simulink model "off_grid_NPC"  (R2015b)
settings: Solver=ode23tb  StartTime=0.0  StopTime=4  RelTol=1e-3
PreLoadFcn:
  | load  power_3levelVSC.mat
  | Ts_Power=5e-6;
  | Ts_Control=100e-6;
undefined symbols (not defined in the file): DiscIntNeverNeededParam
libraries: powerlib x25, powerlib_meascontrol x18, powerlib_extras x6, simulink x6, simulink_extras x1
settings Model: Creator=Pouyan  LastModifiedBy=fujitsu
settings DataIOCC: SaveFormat=Array  SignalLoggingSaveFormat=ModelDataLogs
settings OptimizationCC: ExpressionDepthLimit=2147483647
settings DebuggingCC: UnderspecifiedInitializationDetection=Classic  MergeDetectMultiDrivingBlocksExec=none  SolverPrmCheckMsg=warning  FcnCallInpInsideContextMsg=UseLocalSettings  StateNameClashWarn=warning
settings HardwareCC: ProdBitPerPointer=32  ProdLargestAtomicFloat=None  ProdIntDivRoundTo=Undefined  ProdEndianess=Unspecified  ProdWordSize=32  ProdHWDeviceType=32-bit Generic
settings GRTTargetCC: GeneratePreprocessorConditionals=Disable all  CombineOutputUpdateFcns=off  GRTInterface=on
settings ConfigComp: CovModelRefEnable=Off

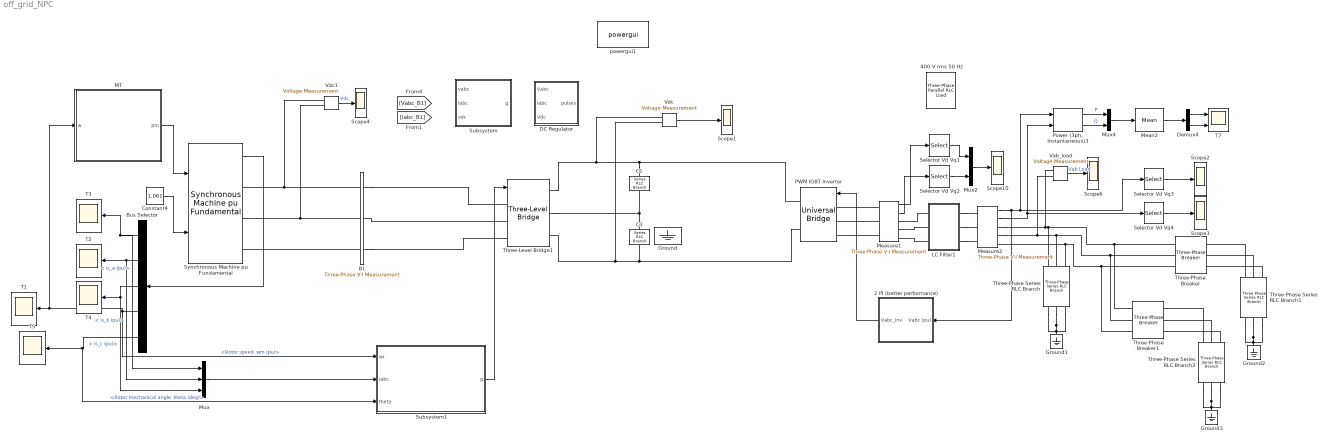
== system off_grid_NPC ==
  " 400 V rms 50 Hz" : powerlib/Elements/Three-Phase Parallel RLC Load  LConnTagsString=A|B|C  Configuration=Y (grounded)  NominalVoltage=400  Vabc=[1e3 1e3 1e3]  Vabcp=[1e3 1e3 1e3]  NominalFrequency=50  UnbalancedPower=off  ActivePower=50e3  InductivePower=0  CapacitivePower=0  Pabc=[10e3 9e3 11e3]  QLabc=[100 90 110]  QCabc=[100 90 110]  Pabcp=[10e3 9e3 11e3]  QLabcp=[100 90 110]  QCabcp=[100 90 110]  Measurements=None  LoadType=constant Z
  2 PI (better performance) : Subsystem  mask{kp=0.01, ki=5}
  B1 : powerlib/Measurements/Three-Phase V-I Measurement  VoltageMeasurement=phase-to-ground  SetLabelV=on  LabelV=Vabc_B1  Vpu=off  VpuLL=off  CurrentMeasurement=yes  SetLabelI=on  LabelI=Iabc_B1  Ipu=off  Pbase=100e6  Vbase=500e3  OutputType=Magnitude  PhasorSimulation=off  PSBequivalent=0
  Bus Selector : BusSelector  OutputSignals="Stator current. is_a (pu),Stator current. is_b (pu),Stator current. is_c (pu),Mechanical.Rotor speed  wm (pu),Mechanical.Rotor mechanical angle  theta (deg)"
  C1 : powerlib/Elements/Series RLC Branch  LConnTagsString=__new0  RConnTagsString=__new0  BranchType=C  Resistance=1.0  Inductance=1.0  SetiL0=off  InitialCurrent=0  Capacitance=75000e-06  Setx0=off  InitialVoltage=0  Measurements=None
  C3 : powerlib/Elements/Series RLC Branch  LConnTagsString=__new0  RConnTagsString=__new0  BranchType=C  Resistance=1.0  Inductance=1.0  SetiL0=off  InitialCurrent=0  Capacitance=75000e-06  Setx0=off  InitialVoltage=0  Measurements=None
  Constant4 : Constant  Value=1.061
  DC Regulator : Subsystem  mask(DC Voltage Regulator){Vdc_Ref=750}
      mask prompts: Vdc_Ref "DC voltage setpoint (V):"
  Demux4 : Demux  Outputs=2
  Ground{,1..3} (4 alike) : powerlib/Elements/Ground  LConnTagsString=a
  LC Filter1 : Subsystem
  MT : Subsystem
  Mean2 : powerlib_meascontrol/Measurements/Mean  Freq=50  Vinit=0  Ts=50e-6
  Measure1 : powerlib/Measurements/Three-Phase V-I Measurement  VoltageMeasurement=phase-to-phase  SetLabelV=off  LabelV=V1  Vpu=off  VpuLL=off  CurrentMeasurement=yes  SetLabelI=off  LabelI=I1  Ipu=off  Pbase=10e3  Vbase=400  OutputType=Magnitude  PhasorSimulation=off  PSBequivalent=0
  Measure2 : powerlib/Measurements/Three-Phase V-I Measurement  VoltageMeasurement=phase-to-phase  SetLabelV=off  LabelV=V1  Vpu=off  VpuLL=on  CurrentMeasurement=yes  SetLabelI=off  LabelI=I1  Ipu=on  Pbase=20e3  Vbase=400  OutputType=Magnitude  PhasorSimulation=off  PSBequivalent=0
  Mux : Mux  Inputs=3
  Mux2 : Mux  Inputs=2
  Mux4 : Mux  Inputs=2
  PWM IGBT Inverter : powerlib/Power Electronics/Universal Bridge  Arms=3  SnubberResistance=5000  SnubberCapacitance=inf  Device=IGBT / Diodes  Ron=1e-3  Lon=0  ForwardVoltages="[  0.0  0.0  ]"  ForwardVoltage=.8  GTOparameters=[ 1e-6 ,1e-6 ]  IGBTparameters=[ 1e-6 , 2e-6 ]  Measurements=Device currents  Measurements_2=None  converterType=Rectifier
  "Power (3ph, Instantaneous)3" : powerlib_meascontrol/Measurements/Power (3ph, Instantaneous)
  Scope{1..4,6,10} (6 alike) : Scope
  Selector Vd Vq{1..4} (4 alike) : Selector  InputPortWidth=3  IndexOptions=Index vector (dialog)  Indices=[1]  OutputSizes=1
  Subsystem : Subsystem  mask{kp=1, ki=5, dcref=750}
      mask prompts: dcref "Vdc_ref"
  Subsystem1 : Subsystem  mask{kp=1, ki=5}
  Synchronous Machine pu Fundamental : powerlib/Machines/Synchronous Machine pu Fundamental  PresetModel=No  MechanicalLoad=Mechanical power Pm  ShowDetailedParameters=on  RotorType=Salient-pole  Units=per unit fundamental parameters  MeasurementBus=off  NominalParameters="[ 60e3  500 1600]"  Stator="[ 0.2503  0.114  0.6875  0.6875 ]"  Field="[ 1  10e15/(100*pi)]"  Dampers2=[0.0652, 0.5134, 0.0287, 0.2553, 7.765e-3, 0.9167 ]  Dampers1="[ 1.17E-02  0.182  1.97E-02  0.384 ]"  Mechanical=[ 6 0 2]  PolePairs=20  InitialConditions="[ 0  0  0  0  0  0  0  0  1 ]"  SetSaturation=off  Saturation=[0.6404,0.7127,0.8441,0.9214,0.9956,1.082,1.19,1.316,1.457;0.7,0.7698,0.8872,0.9466,0.9969,1.046,1.1,1.151,1.201]  LoadFlowParameters=[1,0,0,0,0]  TsPowergui=0  TsBlock=-1  IterativeModel=Trapezoidal non iterative  BusType=swing  Pref=0  Qref=0  Qmin=-inf  Qmax=inf  PLF=0  QLF=0
  T{1..5} (5 alike) : Scope
  T7 : Scope  NumInputPorts=2
  Three-Level Bridge1 : powerlib/Power Electronics/Three-Level Bridge  Arms=3  SnubberResistance=100  SbubberCapacitance=1e-6  Device=IGBT / Diodes  Ron=1e-3  ForwardVoltages=[370 1]  Measurements=All voltages and currents
  Three-Phase Series RLC Branch : powerlib/Elements/Three-Phase Series RLC Branch  LConnTagsString=A|B|C  RConnTagsString=A|B|C  BranchType=R  Resistance=400^2/20000  Inductance=1e-3  Capacitance=1e-6  Measurements=None
  Three-Phase Series RLC Branch1 : powerlib/Elements/Three-Phase Series RLC Branch  LConnTagsString=A|B|C  RConnTagsString=A|B|C  BranchType=R  Resistance=400^2/10000  Inductance=1e-3  Capacitance=1e-6  Measurements=None
  Three-Phase Series RLC Branch2 : powerlib/Elements/Three-Phase Series RLC Branch  LConnTagsString=A|B|C  RConnTagsString=A|B|C  BranchType=R  Resistance=400^2/20000  Inductance=1e-3  Capacitance=1e-6  Measurements=None
  Three-Phase Breaker : powerlib/Elements/Three-Phase Breaker  InitialState=open  SwitchA=on  SwitchB=on  SwitchC=on  SwitchTimes=[1 3]  External=off  BreakerResistance=0.01  SnubberResistance=1e6  SnubberCapacitance=inf  Measurements=None
  Three-Phase Breaker1 : powerlib/Elements/Three-Phase Breaker  InitialState=open  SwitchA=on  SwitchB=on  SwitchC=on  SwitchTimes=[2]  External=off  BreakerResistance=0.01  SnubberResistance=1e6  SnubberCapacitance=inf  Measurements=None
  Vab_load : powerlib/Measurements/Voltage Measurement  Tag=PoWeRsYsTeMmEaSuReMeNt  PhasorSimulation=off  OutputType=Magnitude  PSBequivalent=0
  "Vdc " : powerlib/Measurements/Voltage Measurement  Tag=PoWeRsYsTeMmEaSuReMeNt  PhasorSimulation=off  OutputType=Magnitude  PSBequivalent=0
  Vdc1 : powerlib/Measurements/Voltage Measurement  Tag=PoWeRsYsTeMmEaSuReMeNt  PhasorSimulation=off  OutputType=Magnitude  PSBequivalent=0
  powergui1 : powerlib/powergui  Priority=2  SimulationMode=Discrete  SolverType=Tustin/Backward Euler (TBE)  SampleTime=Ts_Power  frequency=60  SPID=off  DisableSnubberDevices=off  DisableRonSwitches=off  DisableVfSwitches=off  SwTol=0  DisplayEquations=off  Interpol=off  ExternalGateDelay=off  methode=off  Ts=0  FunctionMessages=off  echomessages=off  HookPort=off  EnableUseOfTLC=off  x0status=blocks  frequencyindice=0  Pbase=100e6  ErrMax=1e-4  Iterations=50  UnitsV=kV  UnitsW=MW  buscounter=0  RestoreLinks=warning  ResistiveCurrentMeasurement=off  Frange=logspace(0,3,50)  Ylog=off  Xlog=off  ShowGrid=off  save=off  variable=ZData  structure=VaIa  ZoomFFT=on  StartTime=0.2  cycles=2  DisplayStyle=1  fundamental=60  FreqAxis=off  MaxFrequency=1000  frequencyindicesteady=1  RmsSteady=2  display=off
  wires:
  Vab_load/1 -> Scope6/1  "Vab Load"
  Mux4/1 -> Mean2/1
  Mean2/1 -> Demux4/1
  "Power (3ph, Instantaneous)3"/1 -> Mux4/1  "P"
  "Power (3ph, Instantaneous)3"/2 -> Mux4/2  "Q"
  Demux4/1 -> T7/1
  Demux4/2 -> T7/2
  "Vdc "/1 -> Scope1/1
  MT/1(pm) -> Synchronous Machine pu Fundamental/1
  Synchronous Machine pu Fundamental/1 -> Bus Selector/1
  Bus Selector/4 -> Subsystem1/1(wr), MT/1(w), T1/1  "<Rotor speed  wm (pu)>"
  Constant4/1 -> Synchronous Machine pu Fundamental/2
  Vdc1/1 -> Scope4/1  "Vdc"
  Mux2/1 -> Scope10/1
  Measure1/1 -> Selector Vd Vq1/1
  Selector Vd Vq1/1 -> Mux2/1
  Measure1/2 -> Selector Vd Vq2/1
  Selector Vd Vq2/1 -> Mux2/2
  Measure2/1 -> 2 PI (better performance)/1(Vabc (pu)), "Power (3ph, Instantaneous)3"/1, Selector Vd Vq3/1
  Measure2/2 -> "Power (3ph, Instantaneous)3"/2, Selector Vd Vq4/1
  Selector Vd Vq3/1 -> Scope2/1
  Selector Vd Vq4/1 -> Scope3/1
  2 PI (better performance)/1(Vabc_inv) -> PWM IGBT Inverter/1
  Bus Selector/1 -> Mux/1, T3/1  "< is_a (pu)>"
  Bus Selector/2 -> T2/1, Mux/2  "< is_b (pu)>"
  Bus Selector/3 -> Mux/3, T4/1  "< is_c (pu)>"
  Bus Selector/5 -> Subsystem1/3(theta), T5/1  "<Rotor mechanical angle  theta (deg)>"
  Mux/1 -> Subsystem1/2(iabc)
  Subsystem1/1(g) -> Three-Level Bridge1/1
  connections:
  Measure2/RConn2 -- Three-Phase Breaker1/LConn2 -- Three-Phase Breaker/LConn2 -- Three-Phase Series RLC Branch/LConn2 -- Vab_load/LConn2
  Measure2/RConn1 -- Three-Phase Breaker1/LConn1 -- Three-Phase Breaker/LConn1 -- Three-Phase Series RLC Branch/LConn1 -- Vab_load/LConn1
  C3/LConn1 -- C1/RConn1 -- Three-Level Bridge1/RConn2
  C3/RConn1 -- Three-Level Bridge1/RConn3 -- "Vdc "/LConn2 -- PWM IGBT Inverter/RConn2
  C1/LConn1 -- Three-Level Bridge1/RConn1 -- "Vdc "/LConn1 -- PWM IGBT Inverter/RConn1
  B1/RConn1 -- Three-Level Bridge1/LConn1
  B1/RConn3 -- Three-Level Bridge1/LConn3
  Three-Level Bridge1/LConn2 -- B1/RConn2
  B1/LConn1 -- Vdc1/LConn1 -- Synchronous Machine pu Fundamental/RConn1
  B1/LConn2 -- Vdc1/LConn2 -- Synchronous Machine pu Fundamental/RConn2
  B1/LConn3 -- Synchronous Machine pu Fundamental/RConn3
  Three-Phase Series RLC Branch/RConn3 -- Three-Phase Series RLC Branch/RConn2 -- Ground1/LConn1 -- Three-Phase Series RLC Branch/RConn1
  LC Filter1/LConn3 -- Measure1/RConn3
  LC Filter1/RConn3 -- Measure2/LConn3
  LC Filter1/LConn2 -- Measure1/RConn2
  LC Filter1/RConn2 -- Measure2/LConn2
  LC Filter1/LConn1 -- Measure1/RConn1
  LC Filter1/RConn1 -- Measure2/LConn1
  Measure1/LConn1 -- PWM IGBT Inverter/LConn1
  Measure1/LConn2 -- PWM IGBT Inverter/LConn2
  Measure1/LConn3 -- PWM IGBT Inverter/LConn3
  Three-Phase Series RLC Branch/LConn3 -- Three-Phase Breaker1/LConn3 -- Three-Phase Breaker/LConn3 -- Measure2/RConn3
  Three-Phase Series RLC Branch1/RConn3 -- Three-Phase Series RLC Branch1/RConn2 -- Ground2/LConn1 -- Three-Phase Series RLC Branch1/RConn1
  Three-Phase Series RLC Branch1/LConn1 -- Three-Phase Breaker/RConn1
  Three-Phase Series RLC Branch1/LConn2 -- Three-Phase Breaker/RConn2
  Three-Phase Series RLC Branch1/LConn3 -- Three-Phase Breaker/RConn3
  Three-Phase Series RLC Branch2/RConn3 -- Three-Phase Series RLC Branch2/RConn1 -- Three-Phase Series RLC Branch2/RConn2 -- Ground3/LConn1
  Three-Phase Series RLC Branch2/LConn2 -- Three-Phase Breaker1/RConn2
  Three-Phase Series RLC Branch2/LConn3 -- Three-Phase Breaker1/RConn3
  Three-Phase Series RLC Branch2/LConn1 -- Three-Phase Breaker1/RConn1

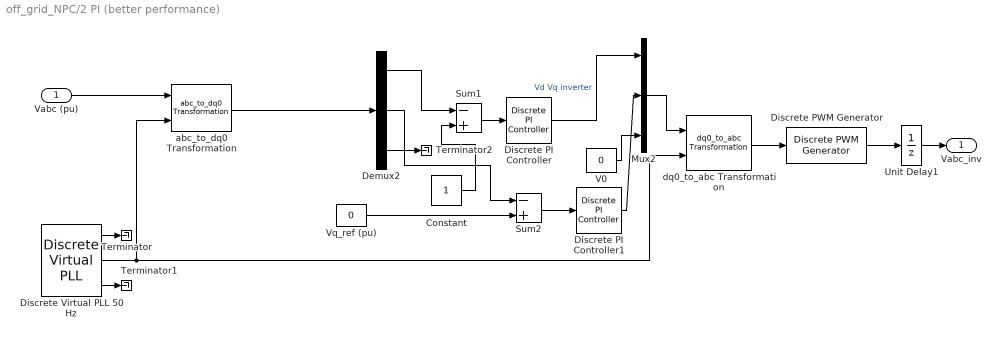
== system off_grid_NPC/2 PI (better performance) ==
  Vabc (pu) : Inport
  Constant : Constant
  Demux2 : Demux  Outputs=3
  Discrete PI Controller : powerlib_extras/Discrete  Control Blocks/Discrete PI Controller  Kp=kp  Ki=ki  Par_Limits=[1 -1]  Init=0  Ts=5e-6
  Discrete PI Controller1 : powerlib_extras/Discrete  Control Blocks/Discrete PI Controller  Kp=kp  Ki=ki  Par_Limits=[1 -1]  Init=0  Ts=5e-6
  Discrete PWM Generator : powerlib_extras/Discrete  Control Blocks/Discrete PWM Generator  GeneratorMode="3-arm  bridge (6 pulses)"  Fc=2000  Ts=5e-6  Internal=off  mIndex=0.4  Freq=60  Phase=0
  Discrete Virtual PLL 50 Hz : powerlib_extras/Discrete  Control Blocks/Discrete Virtual PLL  Freq=50  Phase=0  Ts=5e-6
  Mux2 : Mux  Inputs=3
  Sum1 : Sum  Inputs=-+  SaturateOnIntegerOverflow=on  InputSameDT=on  OutDataTypeStr=Inherit: Same as first input
  Sum2 : Sum  Inputs=-+  SaturateOnIntegerOverflow=on  InputSameDT=on  OutDataTypeStr=Inherit: Same as first input
  Terminator : Terminator
  Terminator1 : Terminator
  Terminator2 : Terminator
  Unit Delay1 : UnitDelay  SampleTime=2e-6
  V0 : Constant  Value=0
  Vq_ref (pu) : Constant  Value=0
  abc_to_dq0 Transformation : powerlib_extras/Measurements/abc_to_dq0 Transformation
  dq0_to_abc Transformation : powerlib_extras/Measurements/dq0_to_abc Transformation
  Vabc_inv : Outport
  wires:
  Vabc (pu)/1 -> abc_to_dq0 Transformation/1
  Demux2/1 -> Sum1/1
  Sum1/1 -> Discrete PI Controller/1
  Mux2/1 -> dq0_to_abc Transformation/1
  Discrete Virtual PLL 50 Hz/2 -> abc_to_dq0 Transformation/2, dq0_to_abc Transformation/2
  Discrete Virtual PLL 50 Hz/1 -> Terminator/1
  Discrete Virtual PLL 50 Hz/3 -> Terminator1/1
  Discrete PWM Generator/1 -> Unit Delay1/1
  dq0_to_abc Transformation/1 -> Discrete PWM Generator/1
  Unit Delay1/1 -> Vabc_inv/1
  abc_to_dq0 Transformation/1 -> Demux2/1
  Demux2/3 -> Terminator2/1
  Constant/1 -> Sum1/2
  Demux2/2 -> Sum2/1
  Vq_ref (pu)/1 -> Sum2/2
  Sum2/1 -> Discrete PI Controller1/1
  Discrete PI Controller/1 -> Mux2/1  "Vd Vq inverter"
  Discrete PI Controller1/1 -> Mux2/2
  V0/1 -> Mux2/3

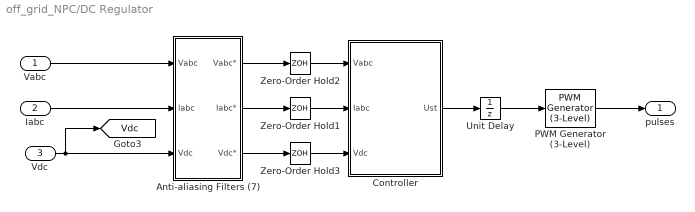
== system off_grid_NPC/DC Regulator ==
  Vabc : Inport  PortDimensions=3
  Iabc : Inport  Port=2  PortDimensions=3
  Vdc : Inport  Port=3  PortDimensions=1
  Anti-aliasing Filters (7) : Subsystem  mask(Anti-aliasing (2nd order lowpass)){Fc=5000, Ts=Ts_Power}
      mask prompts: Fc "Cut-off frequency (Hz):"; Ts "Sample time:"
  Controller : Subsystem  mask(DC Regulator){Vdc_Ref=Vdc_Ref, Par_VdcReg=[0.015 1.6], Par_IReg=[0.3 20], Par_Nom=[600 500e3], Ts=Ts_Control}
      mask prompts: Vdc_Ref "DC Voltage setpoint (Volts)"; Par_VdcReg "Vdc Regulator Gains: [ Kp  Ki ]"; Par_IReg "Current Regulators Gain: [ Kp Ki Kd ]"; Par_Nom "Nominal Voltage and power: [ Vnom (volts rms L-L)  Pnom (VA) ]"; Ts "Time Step (s)"
      mask init:
      | Vnom=Par_Nom(1);
      | Pnom=Par_Nom(2);
      | Kp_I=Par_IReg(1);
      | Ki_I=Par_IReg(2);
      | Kp_Vdc=Par_VdcReg(1);
      | Ki_Vdc=Par_VdcReg(2);
  PWM Generator (3-Level) : powerlib_meascontrol/Pulse & Signal Generators/PWM Generator (3-Level)  ModulatorType=Three-phase bridge (12 pulses)  ModulatorMode=Unsynchronized  nF=27  Fc=50*1000  ModulatingSignals=off  m=0.8  Freq=60  Phase=0  Ts=Ts_Power
  Unit Delay : UnitDelay  SampleTime=Ts_Control
  Zero-Order Hold1 : ZeroOrderHold  SampleTime=Ts_Control
  Zero-Order Hold2 : ZeroOrderHold  SampleTime=Ts_Control
  Zero-Order Hold3 : ZeroOrderHold  SampleTime=Ts_Control
  pulses : Outport
  tag scope: Vdc=global
  wires:
  PWM Generator (3-Level)/1 -> pulses/1
  Unit Delay/1 -> PWM Generator (3-Level)/1
  Controller/1(Ust) -> Unit Delay/1
  Anti-aliasing Filters (7)/1(" Vabc*") -> Zero-Order Hold2/1
  Anti-aliasing Filters (7)/2(Iabc*) -> Zero-Order Hold1/1
  Anti-aliasing Filters (7)/3(" Vdc*") -> Zero-Order Hold3/1
  Zero-Order Hold3/1 -> Controller/3(Vdc)
  Zero-Order Hold1/1 -> Controller/2(Iabc)
  Zero-Order Hold2/1 -> Controller/1(Vabc)
  Vdc/1 -> [Vdc], Anti-aliasing Filters (7)/3("Vdc ")
  Iabc/1 -> Anti-aliasing Filters (7)/2("Iabc ")
  Vabc/1 -> Anti-aliasing Filters (7)/1(Vabc)

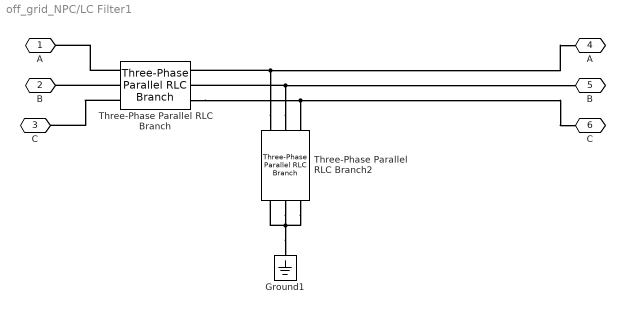
== system off_grid_NPC/LC Filter1 ==
  Ground1 : powerlib/Elements/Ground  LConnTagsString=a
  Three-Phase Parallel RLC Branch : powerlib/Elements/Three-Phase Parallel RLC Branch  LConnTagsString=A|B|C  RConnTagsString=A|B|C  BranchType=L  Resistance=1  Inductance=5.7e-3  Capacitance=1e-6  Measurements=None
  Three-Phase Parallel RLC Branch2 : powerlib/Elements/Three-Phase Parallel RLC Branch  LConnTagsString=A|B|C  RConnTagsString=A|B|C  BranchType=C  Resistance=1  Inductance=5.7e-3  Capacitance=1000e-6  Measurements=None
  A : PMIOPort  Port=1  Side=Left
  B : PMIOPort  Port=2  Side=Left
  C : PMIOPort  Port=3  Side=Left
  "A " : PMIOPort  Port=4  Side=Right
  "B " : PMIOPort  Port=5  Side=Right
  "C " : PMIOPort  Port=6  Side=Right
  connections:
  Ground1/LConn1 -- Three-Phase Parallel RLC Branch2/RConn2 -- Three-Phase Parallel RLC Branch2/RConn1 -- Three-Phase Parallel RLC Branch2/RConn3
  Three-Phase Parallel RLC Branch/RConn3 -- Three-Phase Parallel RLC Branch2/LConn3 -- "C "/RConn1
  Three-Phase Parallel RLC Branch2/LConn2 -- "B "/RConn1 -- Three-Phase Parallel RLC Branch/RConn2
  Three-Phase Parallel RLC Branch2/LConn1 -- "A "/RConn1 -- Three-Phase Parallel RLC Branch/RConn1
  Three-Phase Parallel RLC Branch/LConn3 -- C/RConn1
  Three-Phase Parallel RLC Branch/LConn2 -- B/RConn1
  Three-Phase Parallel RLC Branch/LConn1 -- A/RConn1

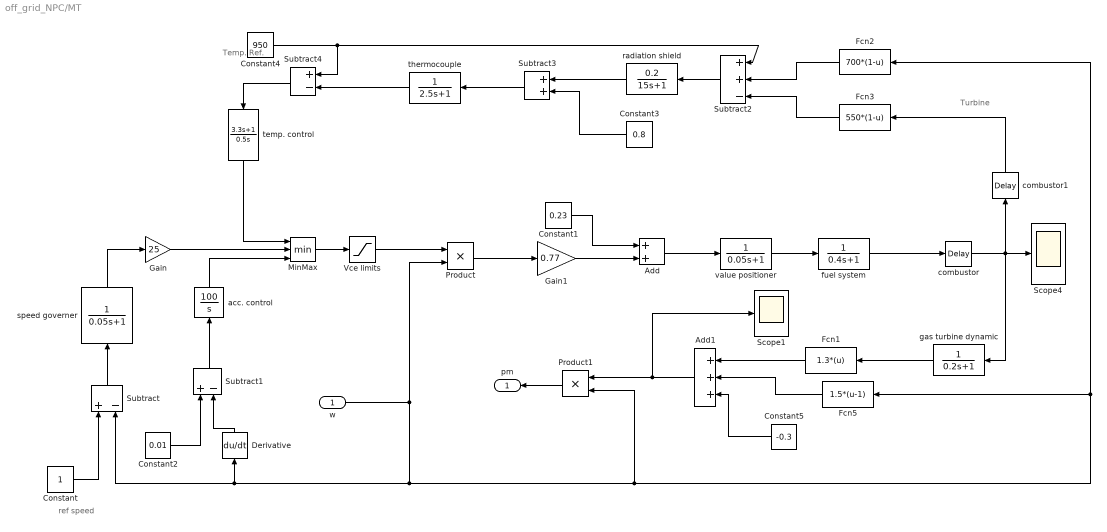
== system off_grid_NPC/MT ==
  note: ref speed
  note: Temp.
      | Ref.
  note: Turbine
  w : Inport
  Add : Sum
  Add1 : Sum  Inputs=+++
  Constant : Constant
  Constant1 : Constant  Value=0.23
  Constant2 : Constant  Value=0.01
  Constant3 : Constant  Value=0.8
  Constant4 : Constant  Value=950
  Constant5 : Constant  Value=-0.3
  Derivative : Derivative  CoefficientInTFapproximation=0.001
  Fcn1 : Fcn  Expr=1.3*(u)
  Fcn2 : Fcn  Expr=700*(1-u)
  Fcn3 : Fcn  Expr=550*(1-u)
  Fcn5 : Fcn  Expr=1.5*(u-1)
  Gain : Gain  Gain=25
  Gain1 : Gain  Gain=0.77
  MinMax : MinMax  Inputs=3
  Product : Product  RndMeth=Zero
  Product1 : Product  RndMeth=Zero
  Scope1 : Scope
  Scope4 : Scope
  Subtract : Sum  Inputs=+-
  Subtract1 : Sum  Inputs=+-
  Subtract2 : Sum  Inputs=++-
  Subtract3 : Sum
  Subtract4 : Sum  Inputs=+-
  Vce limits : Saturate  UpperLimit=1.5  LowerLimit=-0.1
  acc. control : TransferFcn  Numerator=[0 100]  Denominator=[1 0]
  combustor : TransportDelay  DelayTime=0.01
  combustor1 : TransportDelay  DelayTime=0.04
  fuel system : TransferFcn  Denominator=[0.4 1]
  gas turbine dynamic : TransferFcn  Denominator=[0.2 1]
  radiation shield : TransferFcn  Numerator=[0.2]  Denominator=[15 1]
  speed governer : TransferFcn  Numerator=[0 1]  Denominator=[0.05 1]
  temp. control : TransferFcn  Numerator=[3.3 1]  Denominator=[0.5 0]
  thermocouple : TransferFcn  Denominator=[2.5 1]
  value positioner : TransferFcn  Denominator=[0.05 1]
  pm : Outport
  wires:
  Constant/1 -> Subtract/1
  Subtract/1 -> speed governer/1
  Vce limits/1 -> Product/1
  Product/1 -> Gain1/1
  Gain1/1 -> Add/2
  Constant1/1 -> Add/1
  Add/1 -> value positioner/1
  value positioner/1 -> fuel system/1
  fuel system/1 -> combustor/1
  combustor/1 -> gas turbine dynamic/1, combustor1/1, Scope4/1
  Add1/1 -> Scope1/1, Product1/1
  Gain/1 -> MinMax/2
  Derivative/1 -> Subtract1/2
  Constant2/1 -> Subtract1/1
  Subtract1/1 -> acc. control/1
  acc. control/1 -> MinMax/3
  MinMax/1 -> Vce limits/1
  combustor1/1 -> Fcn3/1
  Fcn3/1 -> Subtract2/3
  Fcn2/1 -> Subtract2/2
  radiation shield/1 -> Subtract3/1
  Constant3/1 -> Subtract3/2
  Subtract2/1 -> radiation shield/1
  Subtract3/1 -> thermocouple/1
  thermocouple/1 -> Subtract4/2
  Constant4/1 -> Subtract4/1, Subtract2/1
  Subtract4/1 -> temp. control/1
  temp. control/1 -> MinMax/1
  speed governer/1 -> Gain/1
  w/1 -> Product/2, Product1/2, Fcn2/1, Fcn5/1, Derivative/1, Subtract/2
  gas turbine dynamic/1 -> Fcn1/1
  Fcn1/1 -> Add1/1
  Constant5/1 -> Add1/3
  Fcn5/1 -> Add1/2
  Product1/1 -> pm/1

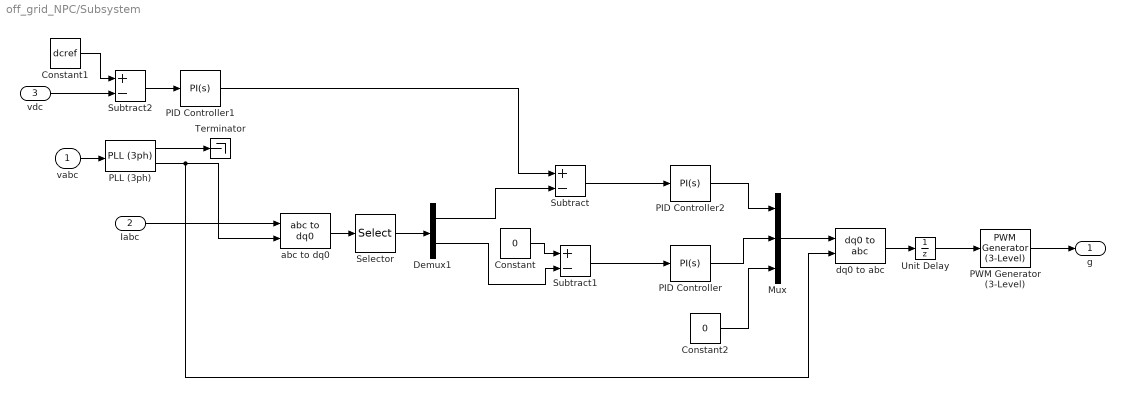
== system off_grid_NPC/Subsystem ==
  vabc : Inport
  Iabc : Inport  Port=2
  vdc : Inport  Port=3
  Constant : Constant  Value=0
  Constant1 : Constant  Value=dcref
  Constant2 : Constant  Value=0
  Demux1 : Demux  Outputs=2
  Mux : Mux  Inputs=3
  PID Controller : simulink/Continuous/PID Controller  Controller=PI  TimeDomain=Continuous-time  SampleTime=-1  IntegratorMethod=Forward Euler  FilterMethod=Forward Euler  Form=Parallel  UseFilter=on  ControllerParametersSource=internal  P=kp  I=ki  D=0  N=100  InitialConditionSource=internal  InitialConditionForIntegrator=0  InitialConditionForFilter=0  ExternalReset=none  LimitOutput=off  UpperSaturationLimit=inf  LowerSaturationLimit=-inf  LinearizeAsGain=on  AntiWindupMode=none  Kb=1  TrackingMode=off  Kt=1  PParamMin=[]  PParamMax=[]  IParamMin=[]  IParamMax=[]  DParamMin=[]  DParamMax=[]  NParamMin=[]  NParamMax=[]  KbParamMin=[]  KbParamMax=[]  KtParamMin=[]  KtParamMax=[]  POutMin=[]  POutMax=[]  IOutMin=[]  IOutMax=[]  DOutMin=[]  DOutMax=[]  NOutMin=[]  NOutMax=[]  KbOutMin=[]  KbOutMax=[]  KtOutMin=[]  KtOutMax=[]  IntegratorOutMin=[]  IntegratorOutMax=[]  FilterOutMin=[]  FilterOutMax=[]  SumOutMin=[]  SumOutMax=[]  SumI1OutMin=[]  SumI1OutMax=[]  SumI2OutMin=[]  SumI2OutMax=[]  SumI3OutMin=[]  SumI3OutMax=[]  SumDOutMin=[]  SumDOutMax=[]  SaturationOutMin=[]  SaturationOutMax=[]  IntegratorContinuousStateAttributes=''  IntegratorStateMustResolveToSignalObject=off  IntegratorRTWStateStorageClass=Auto  FilterContinuousStateAttributes=''  FilterStateMustResolveToSignalObject=off  FilterRTWStateStorageClass=Auto  DifferentiatorICPrevScaledInput=0  DifferentiatorOutMin=[]  DifferentiatorOutMax=[]
  PID Controller1 : simulink/Continuous/PID Controller  Controller=PI  TimeDomain=Continuous-time  SampleTime=-1  IntegratorMethod=Forward Euler  FilterMethod=Forward Euler  Form=Parallel  UseFilter=on  ControllerParametersSource=internal  P=kp  I=ki  D=0  N=100  InitialConditionSource=internal  InitialConditionForIntegrator=0  InitialConditionForFilter=0  ExternalReset=none  LimitOutput=off  UpperSaturationLimit=inf  LowerSaturationLimit=-inf  LinearizeAsGain=on  AntiWindupMode=none  Kb=1  TrackingMode=off  Kt=1  PParamMin=[]  PParamMax=[]  IParamMin=[]  IParamMax=[]  DParamMin=[]  DParamMax=[]  NParamMin=[]  NParamMax=[]  KbParamMin=[]  KbParamMax=[]  KtParamMin=[]  KtParamMax=[]  POutMin=[]  POutMax=[]  IOutMin=[]  IOutMax=[]  DOutMin=[]  DOutMax=[]  NOutMin=[]  NOutMax=[]  KbOutMin=[]  KbOutMax=[]  KtOutMin=[]  KtOutMax=[]  IntegratorOutMin=[]  IntegratorOutMax=[]  FilterOutMin=[]  FilterOutMax=[]  SumOutMin=[]  SumOutMax=[]  SumI1OutMin=[]  SumI1OutMax=[]  SumI2OutMin=[]  SumI2OutMax=[]  SumI3OutMin=[]  SumI3OutMax=[]  SumDOutMin=[]  SumDOutMax=[]  SaturationOutMin=[]  SaturationOutMax=[]  IntegratorContinuousStateAttributes=''  IntegratorStateMustResolveToSignalObject=off  IntegratorRTWStateStorageClass=Auto  FilterContinuousStateAttributes=''  FilterStateMustResolveToSignalObject=off  FilterRTWStateStorageClass=Auto  DifferentiatorICPrevScaledInput=0  DifferentiatorOutMin=[]  DifferentiatorOutMax=[]
  PID Controller2 : simulink/Continuous/PID Controller  Controller=PI  TimeDomain=Continuous-time  SampleTime=-1  IntegratorMethod=Forward Euler  FilterMethod=Forward Euler  Form=Parallel  UseFilter=on  ControllerParametersSource=internal  P=kp  I=ki  D=0  N=100  InitialConditionSource=internal  InitialConditionForIntegrator=0  InitialConditionForFilter=0  ExternalReset=none  LimitOutput=off  UpperSaturationLimit=inf  LowerSaturationLimit=-inf  LinearizeAsGain=on  AntiWindupMode=none  Kb=1  TrackingMode=off  Kt=1  PParamMin=[]  PParamMax=[]  IParamMin=[]  IParamMax=[]  DParamMin=[]  DParamMax=[]  NParamMin=[]  NParamMax=[]  KbParamMin=[]  KbParamMax=[]  KtParamMin=[]  KtParamMax=[]  POutMin=[]  POutMax=[]  IOutMin=[]  IOutMax=[]  DOutMin=[]  DOutMax=[]  NOutMin=[]  NOutMax=[]  KbOutMin=[]  KbOutMax=[]  KtOutMin=[]  KtOutMax=[]  IntegratorOutMin=[]  IntegratorOutMax=[]  FilterOutMin=[]  FilterOutMax=[]  SumOutMin=[]  SumOutMax=[]  SumI1OutMin=[]  SumI1OutMax=[]  SumI2OutMin=[]  SumI2OutMax=[]  SumI3OutMin=[]  SumI3OutMax=[]  SumDOutMin=[]  SumDOutMax=[]  SaturationOutMin=[]  SaturationOutMax=[]  IntegratorContinuousStateAttributes=''  IntegratorStateMustResolveToSignalObject=off  IntegratorRTWStateStorageClass=Auto  FilterContinuousStateAttributes=''  FilterStateMustResolveToSignalObject=off  FilterRTWStateStorageClass=Auto  DifferentiatorICPrevScaledInput=0  DifferentiatorOutMin=[]  DifferentiatorOutMax=[]
  PLL (3ph) : powerlib_meascontrol/PLL/PLL (3ph)  Fmin=45  Par_Init=[0, 50]  ParK=[180, 3200, 1]  TcD=1e-4  MaxRateChangeFreq=12  FilterCutOffFreq=25  Ts=0  AGC=on
  PWM Generator (3-Level) : powerlib_meascontrol/Pulse & Signal Generators/PWM Generator (3-Level)  ModulatorType=Three-phase bridge (12 pulses)  ModulatorMode=Unsynchronized  nF=27  Fc=1e3  ModulatingSignals=off  m=0.8  Freq=60  Phase=0  Ts=Ts_Power
  Selector : Selector  InputPortWidth=3  IndexOptions=Index vector (dialog)  Indices=[1 2]  OutputSizes=1
  Subtract : Sum  Inputs=+-
  Subtract1 : Sum  Inputs=+-
  Subtract2 : Sum  Inputs=+-
  Terminator : Terminator
  Unit Delay : UnitDelay  SampleTime=Ts_Control
  abc to dq0 : powerlib_meascontrol/Transformations/abc to dq0  Alignment=90 degrees behind phase A axis
  dq0 to abc : powerlib_meascontrol/Transformations/dq0 to abc  Alignment=90 degrees behind phase A axis
  g : Outport
  wires:
  vabc/1 -> PLL (3ph)/1
  PLL (3ph)/2 -> dq0 to abc/2, abc to dq0/2
  Iabc/1 -> abc to dq0/1
  PLL (3ph)/1 -> Terminator/1
  abc to dq0/1 -> Selector/1
  Selector/1 -> Demux1/1
  Demux1/1 -> Subtract/2
  Demux1/2 -> Subtract1/2
  Constant/1 -> Subtract1/1
  Subtract1/1 -> PID Controller/1
  vdc/1 -> Subtract2/2
  Constant1/1 -> Subtract2/1
  Subtract2/1 -> PID Controller1/1
  PID Controller1/1 -> Subtract/1
  Subtract/1 -> PID Controller2/1
  PID Controller2/1 -> Mux/1
  PID Controller/1 -> Mux/2
  Constant2/1 -> Mux/3
  Mux/1 -> dq0 to abc/1
  dq0 to abc/1 -> Unit Delay/1
  PWM Generator (3-Level)/1 -> g/1
  Unit Delay/1 -> PWM Generator (3-Level)/1

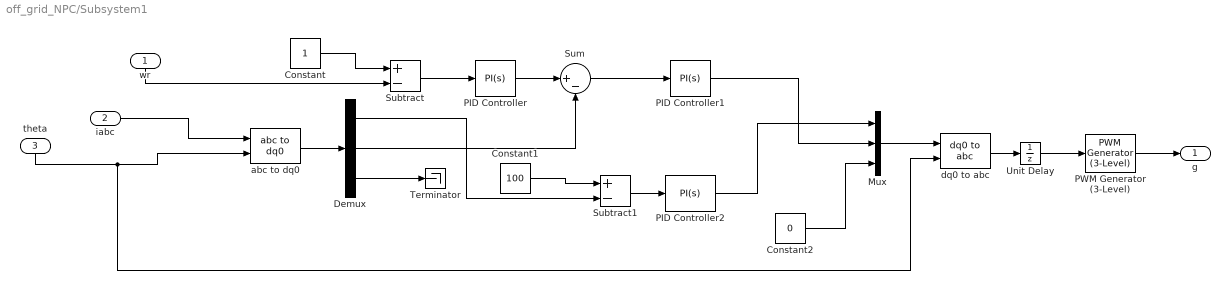
== system off_grid_NPC/Subsystem1 ==
  wr : Inport
  iabc : Inport  Port=2
  theta : Inport  Port=3
  Constant : Constant
  Constant1 : Constant  Value=100
  Constant2 : Constant  Value=0
  Demux : Demux  Outputs=3
  Mux : Mux  Inputs=3
  PID Controller : simulink/Continuous/PID Controller  Controller=PI  TimeDomain=Continuous-time  SampleTime=-1  IntegratorMethod=Forward Euler  FilterMethod=Forward Euler  Form=Parallel  UseFilter=on  ControllerParametersSource=internal  P=kp  I=ki  D=0  N=100  InitialConditionSource=internal  InitialConditionForIntegrator=0  InitialConditionForFilter=0  ExternalReset=none  LimitOutput=off  UpperSaturationLimit=inf  LowerSaturationLimit=-inf  LinearizeAsGain=on  AntiWindupMode=none  Kb=1  TrackingMode=off  Kt=1  PParamMin=[]  PParamMax=[]  IParamMin=[]  IParamMax=[]  DParamMin=[]  DParamMax=[]  NParamMin=[]  NParamMax=[]  KbParamMin=[]  KbParamMax=[]  KtParamMin=[]  KtParamMax=[]  POutMin=[]  POutMax=[]  IOutMin=[]  IOutMax=[]  DOutMin=[]  DOutMax=[]  NOutMin=[]  NOutMax=[]  KbOutMin=[]  KbOutMax=[]  KtOutMin=[]  KtOutMax=[]  IntegratorOutMin=[]  IntegratorOutMax=[]  FilterOutMin=[]  FilterOutMax=[]  SumOutMin=[]  SumOutMax=[]  SumI1OutMin=[]  SumI1OutMax=[]  SumI2OutMin=[]  SumI2OutMax=[]  SumI3OutMin=[]  SumI3OutMax=[]  SumDOutMin=[]  SumDOutMax=[]  SaturationOutMin=[]  SaturationOutMax=[]  IntegratorContinuousStateAttributes=''  IntegratorStateMustResolveToSignalObject=off  IntegratorRTWStateStorageClass=Auto  FilterContinuousStateAttributes=''  FilterStateMustResolveToSignalObject=off  FilterRTWStateStorageClass=Auto  DifferentiatorICPrevScaledInput=0  DifferentiatorOutMin=[]  DifferentiatorOutMax=[]
  PID Controller1 : simulink/Continuous/PID Controller  Controller=PI  TimeDomain=Continuous-time  SampleTime=-1  IntegratorMethod=Forward Euler  FilterMethod=Forward Euler  Form=Parallel  UseFilter=on  ControllerParametersSource=internal  P=kp  I=ki  D=0  N=100  InitialConditionSource=internal  InitialConditionForIntegrator=0  InitialConditionForFilter=0  ExternalReset=none  LimitOutput=off  UpperSaturationLimit=inf  LowerSaturationLimit=-inf  LinearizeAsGain=on  AntiWindupMode=none  Kb=1  TrackingMode=off  Kt=1  PParamMin=[]  PParamMax=[]  IParamMin=[]  IParamMax=[]  DParamMin=[]  DParamMax=[]  NParamMin=[]  NParamMax=[]  KbParamMin=[]  KbParamMax=[]  KtParamMin=[]  KtParamMax=[]  POutMin=[]  POutMax=[]  IOutMin=[]  IOutMax=[]  DOutMin=[]  DOutMax=[]  NOutMin=[]  NOutMax=[]  KbOutMin=[]  KbOutMax=[]  KtOutMin=[]  KtOutMax=[]  IntegratorOutMin=[]  IntegratorOutMax=[]  FilterOutMin=[]  FilterOutMax=[]  SumOutMin=[]  SumOutMax=[]  SumI1OutMin=[]  SumI1OutMax=[]  SumI2OutMin=[]  SumI2OutMax=[]  SumI3OutMin=[]  SumI3OutMax=[]  SumDOutMin=[]  SumDOutMax=[]  SaturationOutMin=[]  SaturationOutMax=[]  IntegratorContinuousStateAttributes=''  IntegratorStateMustResolveToSignalObject=off  IntegratorRTWStateStorageClass=Auto  FilterContinuousStateAttributes=''  FilterStateMustResolveToSignalObject=off  FilterRTWStateStorageClass=Auto  DifferentiatorICPrevScaledInput=0  DifferentiatorOutMin=[]  DifferentiatorOutMax=[]
  PID Controller2 : simulink/Continuous/PID Controller  Controller=PI  TimeDomain=Continuous-time  SampleTime=-1  IntegratorMethod=Forward Euler  FilterMethod=Forward Euler  Form=Parallel  UseFilter=on  ControllerParametersSource=internal  P=kp  I=ki  D=0  N=100  InitialConditionSource=internal  InitialConditionForIntegrator=0  InitialConditionForFilter=0  ExternalReset=none  LimitOutput=off  UpperSaturationLimit=inf  LowerSaturationLimit=-inf  LinearizeAsGain=on  AntiWindupMode=none  Kb=1  TrackingMode=off  Kt=1  PParamMin=[]  PParamMax=[]  IParamMin=[]  IParamMax=[]  DParamMin=[]  DParamMax=[]  NParamMin=[]  NParamMax=[]  KbParamMin=[]  KbParamMax=[]  KtParamMin=[]  KtParamMax=[]  POutMin=[]  POutMax=[]  IOutMin=[]  IOutMax=[]  DOutMin=[]  DOutMax=[]  NOutMin=[]  NOutMax=[]  KbOutMin=[]  KbOutMax=[]  KtOutMin=[]  KtOutMax=[]  IntegratorOutMin=[]  IntegratorOutMax=[]  FilterOutMin=[]  FilterOutMax=[]  SumOutMin=[]  SumOutMax=[]  SumI1OutMin=[]  SumI1OutMax=[]  SumI2OutMin=[]  SumI2OutMax=[]  SumI3OutMin=[]  SumI3OutMax=[]  SumDOutMin=[]  SumDOutMax=[]  SaturationOutMin=[]  SaturationOutMax=[]  IntegratorContinuousStateAttributes=''  IntegratorStateMustResolveToSignalObject=off  IntegratorRTWStateStorageClass=Auto  FilterContinuousStateAttributes=''  FilterStateMustResolveToSignalObject=off  FilterRTWStateStorageClass=Auto  DifferentiatorICPrevScaledInput=0  DifferentiatorOutMin=[]  DifferentiatorOutMax=[]
  PWM Generator (3-Level) : powerlib_meascontrol/Pulse & Signal Generators/PWM Generator (3-Level)  ModulatorType=Three-phase bridge (12 pulses)  ModulatorMode=Unsynchronized  nF=27  Fc=1e3  ModulatingSignals=off  m=0.8  Freq=60  Phase=0  Ts=Ts_Power
  Subtract : Sum  Inputs=+-
  Subtract1 : Sum  Inputs=+-
  Sum : Sum  Inputs=|+-
  Terminator : Terminator
  Unit Delay : UnitDelay  SampleTime=Ts_Control
  abc to dq0 : powerlib_meascontrol/Transformations/abc to dq0  Alignment=90 degrees behind phase A axis
  dq0 to abc : powerlib_meascontrol/Transformations/dq0 to abc  Alignment=90 degrees behind phase A axis
  g : Outport
  wires:
  Sum/1 -> PID Controller1/1
  Subtract/1 -> PID Controller/1
  Constant/1 -> Subtract/1
  iabc/1 -> abc to dq0/1
  Demux/2 -> Sum/2
  Subtract1/1 -> PID Controller2/1
  theta/1 -> dq0 to abc/2, abc to dq0/2
  wr/1 -> Subtract/2
  Demux/1 -> Subtract1/2
  Constant1/1 -> Subtract1/1
  abc to dq0/1 -> Demux/1
  PID Controller/1 -> Sum/1
  Demux/3 -> Terminator/1
  Constant2/1 -> Mux/3
  PID Controller1/1 -> Mux/2
  PID Controller2/1 -> Mux/1
  Mux/1 -> dq0 to abc/1
  dq0 to abc/1 -> Unit Delay/1
  PWM Generator (3-Level)/1 -> g/1
  Unit Delay/1 -> PWM Generator (3-Level)/1

== system off_grid_NPC/DC Regulator/Anti-aliasing Filters (7) ==
  Vabc : Inport  PortDimensions=3
  "Iabc " : Inport  Port=2  PortDimensions=3
  "Vdc " : Inport  Port=3  PortDimensions=1
  Second-Order Filter : powerlib_meascontrol/Filters/Second-Order Filter  FilterType=Lowpass  Fo=Fc  Zeta=0.707  Ts=Ts  Initialize=off  Vac_Init="[0,  0,  60]"  Vdc_Init=0  PlotResponse=off  FreqRange=[0, 500, 1]
  Second-Order Filter1 : powerlib_meascontrol/Filters/Second-Order Filter  FilterType=Lowpass  Fo=Fc  Zeta=0.707  Ts=Ts  Initialize=off  Vac_Init="[0,  0,  60]"  Vdc_Init=0  PlotResponse=off  FreqRange=[0, 500, 1]
  Second-Order Filter2 : powerlib_meascontrol/Filters/Second-Order Filter  FilterType=Lowpass  Fo=Fc  Zeta=0.707  Ts=Ts  Initialize=off  Vac_Init="[0,  0,  60]"  Vdc_Init=0  PlotResponse=off  FreqRange=[0, 500, 1]
  " Vabc*" : Outport
  Iabc* : Outport  Port=2
  " Vdc*" : Outport  Port=3
  wires:
  Second-Order Filter2/1 -> " Vdc*"/1
  "Vdc "/1 -> Second-Order Filter2/1
  Vabc/1 -> Second-Order Filter/1
  Second-Order Filter/1 -> " Vabc*"/1
  "Iabc "/1 -> Second-Order Filter1/1
  Second-Order Filter1/1 -> Iabc*/1

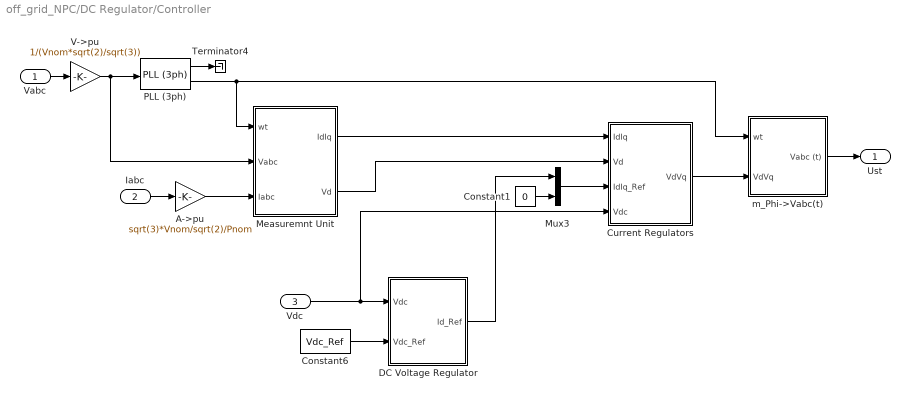
== system off_grid_NPC/DC Regulator/Controller ==
  Vabc : Inport  PortDimensions=3
  Iabc : Inport  Port=2  PortDimensions=3
  Vdc : Inport  Port=3  PortDimensions=1
  A->pu : Gain  Gain=sqrt(3)*Vnom/sqrt(2)/Pnom  SaturateOnIntegerOverflow=on  OutDataTypeStr=Inherit: Same as input  ParamDataTypeStr=Inherit: Same as input
  Constant1 : Constant  Value=0
  Constant6 : Constant  Value=Vdc_Ref
  Current Regulators : Subsystem  mask(Current Regulators){Kp=Kp_I, Ki=Ki_I, Kd=0, TcD=0.2e-3, Par_Limits=[12 -12], Init=0, Ts=Ts}
      mask prompts: Kp "Proportional gain (Kp):"; Ki "Integral gain (Ki):"; Kd "Derivative gain (Kd):"; TcD "Time constant for derivative (s):"; Par_Limits "Output limits: [ Upper   Lower ]"; Init "Output initial value:"; Ts "Sample time:"
      mask help:
      | Sign convention:
      | Id positive(+) flowing into converter ==> Converter absorbing real power = P positive(+)
      | Iq negative(-) flowing into converter (inductive current) ==> Converter absorbing reactive power = Q positive(+)
  DC Voltage Regulator : Subsystem  mask(DC Voltage regulator){Kp=Kp_Vdc, Ki=Ki_Vdc, Ts=Ts}
      mask prompts: Kp "Proportional gain (Kp):"; Ki "Integral gain(Ki)"; Ts "Sample time:"
  Measuremnt Unit : Subsystem
  Mux3 : Mux  Inputs=2
  PLL (3ph) : powerlib_meascontrol/PLL/PLL (3ph)  Fmin=750  Par_Init=[-500 1000]  ParK=[60 1400]  TcD=1e-4  MaxRateChangeFreq=12  FilterCutOffFreq=25  Ts=Ts  AGC=off
  Terminator4 : Terminator
  V->pu : Gain  Gain=1/(Vnom*sqrt(2)/sqrt(3))  SaturateOnIntegerOverflow=on  OutDataTypeStr=Inherit: Same as input  ParamDataTypeStr=Inherit: Same as input
  m_Phi->Vabc(t) : Subsystem
  Ust : Outport
  wires:
  m_Phi->Vabc(t)/1(Vabc (t)) -> Ust/1
  PLL (3ph)/2 -> m_Phi->Vabc(t)/1(wt), Measuremnt Unit/1(wt)
  Current Regulators/1(VdVq) -> m_Phi->Vabc(t)/2(VdVq)
  DC Voltage Regulator/1(Id_Ref) -> Mux3/1
  Constant1/1 -> Mux3/2
  Mux3/1 -> Current Regulators/3(IdIq_Ref)
  Measuremnt Unit/2(Vd) -> Current Regulators/2(Vd)
  Measuremnt Unit/1(IdIq) -> Current Regulators/1(IdIq)
  Iabc/1 -> A->pu/1
  PLL (3ph)/1 -> Terminator4/1
  Vdc/1 -> Current Regulators/4(Vdc), DC Voltage Regulator/1(Vdc)
  Constant6/1 -> DC Voltage Regulator/2(Vdc_Ref)
  Vabc/1 -> V->pu/1
  V->pu/1 -> PLL (3ph)/1, Measuremnt Unit/2(Vabc)
  A->pu/1 -> Measuremnt Unit/3(Iabc)

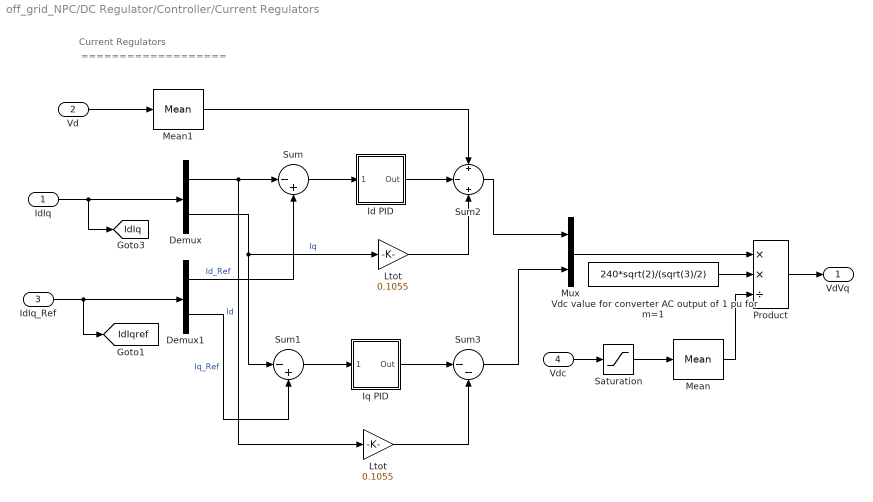
== system off_grid_NPC/DC Regulator/Controller/Current Regulators ==
  note: ===================
  note: Current Regulators
  IdIq : Inport  PortDimensions=2
  Vd : Inport  Port=2
  IdIq_Ref : Inport  Port=3  PortDimensions=2
  Vdc : Inport  Port=4
  " Ltot" : Gain  Gain=0.1055  SaturateOnIntegerOverflow=on  OutDataTypeStr=Inherit: Same as input  ParamDataTypeStr=Inherit: Same as input
  Demux : Demux  Outputs=2
  Demux1 : Demux  Outputs=2
  Id PID : Subsystem  DialogController=POWERSYS.PowerSysDialog  mask(Discrete PID Controller){Kp=Kp, Ki=Ki, Kd=Kd, TcD=TcD, Par_Limits=Par_Limits, Init=Init, Ts=Ts}
      mask prompts: Kp "Proportional gain (Kp):"; Ki "Integral gain (Ki):"; Kd "Derivative gain (Kd):"; TcD "Time constant for derivative (s):"; Par_Limits "Output limits: [ Upper   Lower ]"; Init "Output initial value:"; Ts "Sample time:"
      mask help: This block implements a discrete PID controller.
      mask init:
      | UpperLimit=Par_Limits(1);
      | LowerLimit=Par_Limits(2);
      | power_initmask();
      mask Display: disp('PID');
  Iq PID : Subsystem  DialogController=POWERSYS.PowerSysDialog  mask(Discrete PID Controller){Kp=Kp, Ki=Ki, Kd=Kd, TcD=TcD, Par_Limits=Par_Limits, Init=Init, Ts=Ts}
      mask prompts: Kp "Proportional gain (Kp):"; Ki "Integral gain (Ki):"; Kd "Derivative gain (Kd):"; TcD "Time constant for derivative (s):"; Par_Limits "Output limits: [ Upper   Lower ]"; Init "Output initial value:"; Ts "Sample time:"
      mask help: This block implements a discrete PID controller.
      mask init:
      | UpperLimit=Par_Limits(1);
      | LowerLimit=Par_Limits(2);
      | power_initmask();
      mask Display: disp('PID');
  "Ltot " : Gain  Gain=0.1055  SaturateOnIntegerOverflow=on  OutDataTypeStr=Inherit: Same as input  ParamDataTypeStr=Inherit: Same as input
  Mean : powerlib_meascontrol/Measurements/Mean  Freq=60  Vinit=500  Ts=Ts
  Mean1 : powerlib_meascontrol/Measurements/Mean  Freq=60  Vinit=1.007  Ts=Ts
  Mux : Mux  Inputs=2
  Product : Product  Inputs=**/  SaturateOnIntegerOverflow=on  InputSameDT=on  OutDataTypeStr=Inherit: Same as first input
  Saturation : Saturate  UpperLimit=10000  LowerLimit=10
  Sum : Sum  Inputs=|-+  SaturateOnIntegerOverflow=on  InputSameDT=on  OutDataTypeStr=Inherit: Same as first input
  Sum1 : Sum  Inputs=|-+  SaturateOnIntegerOverflow=on  InputSameDT=on  OutDataTypeStr=Inherit: Same as first input
  Sum2 : Sum  Inputs=+|-|+  SaturateOnIntegerOverflow=on  InputSameDT=on  OutDataTypeStr=Inherit: Same as first input
  Sum3 : Sum  Inputs=|--  SaturateOnIntegerOverflow=on  InputSameDT=on  OutDataTypeStr=Inherit: Same as first input
  Vdc value for converter AC output of 1 pu for m=1 : Constant  Value=240*sqrt(2)/(sqrt(3)/2)
  VdVq : Outport
  tag scope: IdIq=global, IdIqref=global
  wires:
  Sum3/1 -> Mux/2
  Vdc/1 -> Saturation/1
  Mean/1 -> Product/3
  Vdc value for converter AC output of 1 pu for m=1/1 -> Product/2
  Saturation/1 -> Mean/1
  Mean1/1 -> Sum2/1
  Product/1 -> VdVq/1
  IdIq_Ref/1 -> [IdIqref], Demux1/1
  Mux/1 -> Product/1
  Sum/1 -> Id PID/1(Error)
  Demux1/2 -> Sum1/2  "Iq_Ref"
  Sum1/1 -> Iq PID/1(Error)
  Demux/2 -> Sum1/1, "Ltot "/1  "Iq"
  Demux1/1 -> Sum/2  "Id_Ref"
  Demux/1 -> " Ltot"/1, Sum/1  "Id"
  IdIq/1 -> [IdIq], Demux/1
  Id PID/1(Out) -> Sum2/2
  Sum2/1 -> Mux/1
  Iq PID/1(Out) -> Sum3/1
  "Ltot "/1 -> Sum2/3
  " Ltot"/1 -> Sum3/2
  Vd/1 -> Mean1/1

== system off_grid_NPC/DC Regulator/Controller/DC Voltage Regulator ==
  Vdc : Inport
  Vdc_Ref : Inport  Port=2
  -1<Id<+1 : Saturate  UpperLimit=1.2  LowerLimit=-1.2
  Discrete PI Controller : Subsystem  DialogController=POWERSYS.PowerSysDialog  mask(Discrete PI Controller){Kp=Kp, Ki=Ki, Par_Limits=[1.2 -1.2], Init=0, Ts=Ts}
      mask prompts: Kp "Proportional gain (Kp):"; Ki "Integral gain (Ki):"; Par_Limits "Output limits: [ Upper   Lower ]"; Init "Output initial value:"; Ts "Sample time:"
      mask help: This block implements a discrete PI controller.
      mask init:
      | UpperLimit=Par_Limits(1);
      | LowerLimit=Par_Limits(2);
      | power_initmask();
      mask Display: disp('PI');
  Sum : Sum  Inputs=|+-  SaturateOnIntegerOverflow=on  InputSameDT=on  OutDataTypeStr=Inherit: Same as first input
  Id_Ref : Outport  InitialOutput=0
  wires:
  Sum/1 -> Discrete PI Controller/1(Error)
  Vdc/1 -> Sum/2
  Discrete PI Controller/1(Out) -> -1<Id<+1/1
  -1<Id<+1/1 -> Id_Ref/1
  Vdc_Ref/1 -> Sum/1

== system off_grid_NPC/DC Regulator/Controller/Measuremnt Unit ==
  wt : Inport
  Vabc : Inport  Port=2
  Iabc : Inport  Port=3
  Imes : powerlib_meascontrol/Transformations/abc to dq0  Alignment=90 degrees behind phase A axis
  Selector : Selector  InputPortWidth=3  IndexOptions=Index vector (dialog)  Indices=1  OutputSizes=1
  Selector1 : Selector  InputPortWidth=3  IndexOptions=Index vector (dialog)  Indices=[1 2]  OutputSizes=1
  Vmes : powerlib_meascontrol/Transformations/abc to dq0  Alignment=90 degrees behind phase A axis
  IdIq : Outport
  Vd : Outport  Port=2
  wires:
  Selector/1 -> Vd/1
  Imes/1 -> Selector1/1
  Iabc/1 -> Imes/1
  wt/1 -> Imes/2, Vmes/2
  Vmes/1 -> Selector/1
  Vabc/1 -> Vmes/1
  Selector1/1 -> IdIq/1

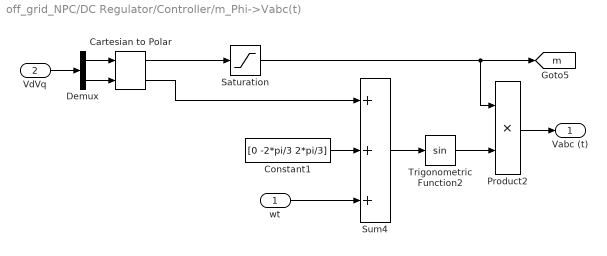
== system off_grid_NPC/DC Regulator/Controller/m_Phi->Vabc(t) ==
  wt : Inport
  VdVq : Inport  Port=2
  Cartesian to Polar : simulink_extras/Transformations/Cartesian to Polar
  Constant1 : Constant  Value=[0 -2*pi/3 2*pi/3]
  Demux : Demux  Outputs=2
  Product2 : Product  SaturateOnIntegerOverflow=on  InputSameDT=on  OutDataTypeStr=Inherit: Same as first input
  Saturation : Saturate  UpperLimit=1  LowerLimit=0
  Sum4 : Sum  Inputs=+++  SaturateOnIntegerOverflow=on  InputSameDT=on  OutDataTypeStr=Inherit: Same as first input
  Trigonometric Function2 : Trigonometry
  Vabc (t) : Outport
  tag scope: m=global
  wires:
  Saturation/1 -> [m], Product2/1
  Cartesian to Polar/1 -> Saturation/1
  Trigonometric Function2/1 -> Product2/2
  Sum4/1 -> Trigonometric Function2/1
  Cartesian to Polar/2 -> Sum4/1
  Demux/2 -> Cartesian to Polar/2
  Demux/1 -> Cartesian to Polar/1
  VdVq/1 -> Demux/1
  wt/1 -> Sum4/3
  Product2/1 -> Vabc (t)/1
  Constant1/1 -> Sum4/2

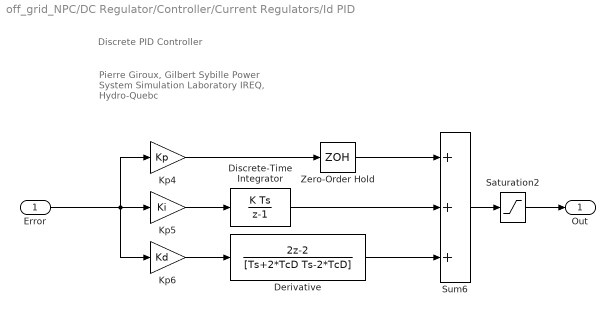
== system off_grid_NPC/DC Regulator/Controller/Current Regulators/Id PID ==
  note: Pierre Giroux, Gilbert Sybille
      | Power System Simulation Laboratory
      | IREQ, Hydro-Quebc
  note: Discrete PID Controller
  Error : Inport  SampleTime=Ts
  "Derivative " : DiscreteTransferFcn  Numerator=[2 -2]  Denominator=[Ts+2*TcD Ts-2*TcD]  SampleTime=Ts
  Discrete-Time Integrator : DiscreteIntegrator  InitialCondition=Init  SampleTime=Ts  LimitOutput=on  UpperSaturationLimit=UpperLimit  LowerSaturationLimit=LowerLimit  ICPrevOutput=DiscIntNeverNeededParam  ICPrevScaledInput=DiscIntNeverNeededParam
  Kp4 : Gain  Gain=Kp  SampleTime=Ts  SaturateOnIntegerOverflow=on  OutDataTypeStr=Inherit: Same as input  ParamDataTypeStr=Inherit: Same as input
  Kp5 : Gain  Gain=Ki  SampleTime=Ts  SaturateOnIntegerOverflow=on  OutDataTypeStr=Inherit: Same as input  ParamDataTypeStr=Inherit: Same as input
  Kp6 : Gain  Gain=Kd  SampleTime=Ts  SaturateOnIntegerOverflow=on  OutDataTypeStr=Inherit: Same as input  ParamDataTypeStr=Inherit: Same as input
  Saturation2 : Saturate  UpperLimit=UpperLimit  LowerLimit=LowerLimit  SampleTime=Ts
  Sum6 : Sum  Inputs=+++  SampleTime=Ts  SaturateOnIntegerOverflow=on  InputSameDT=on  OutDataTypeStr=Inherit: Same as first input
  Zero-Order Hold : ZeroOrderHold  SampleTime=Ts
  Out : Outport  SampleTime=Ts  InitialOutput=0
  wires:
  Saturation2/1 -> Out/1
  Error/1 -> Kp4/1, Kp5/1, Kp6/1
  Sum6/1 -> Saturation2/1
  Kp5/1 -> Discrete-Time Integrator/1
  Kp6/1 -> "Derivative "/1
  Kp4/1 -> Zero-Order Hold/1
  Discrete-Time Integrator/1 -> Sum6/2
  "Derivative "/1 -> Sum6/3
  Zero-Order Hold/1 -> Sum6/1

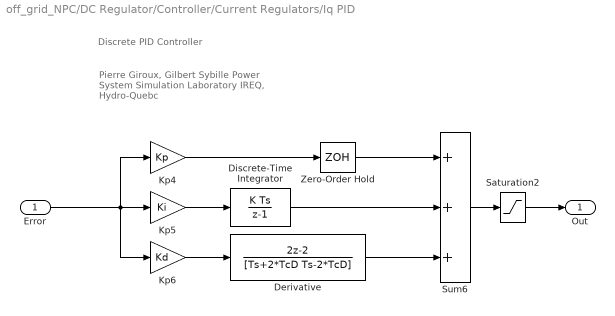
== system off_grid_NPC/DC Regulator/Controller/Current Regulators/Iq PID ==
  note: Pierre Giroux, Gilbert Sybille
      | Power System Simulation Laboratory
      | IREQ, Hydro-Quebc
  note: Discrete PID Controller
  Error : Inport  SampleTime=Ts
  "Derivative " : DiscreteTransferFcn  Numerator=[2 -2]  Denominator=[Ts+2*TcD Ts-2*TcD]  SampleTime=Ts
  Discrete-Time Integrator : DiscreteIntegrator  InitialCondition=Init  SampleTime=Ts  LimitOutput=on  UpperSaturationLimit=UpperLimit  LowerSaturationLimit=LowerLimit  ICPrevOutput=DiscIntNeverNeededParam  ICPrevScaledInput=DiscIntNeverNeededParam
  Kp4 : Gain  Gain=Kp  SampleTime=Ts  SaturateOnIntegerOverflow=on  OutDataTypeStr=Inherit: Same as input  ParamDataTypeStr=Inherit: Same as input
  Kp5 : Gain  Gain=Ki  SampleTime=Ts  SaturateOnIntegerOverflow=on  OutDataTypeStr=Inherit: Same as input  ParamDataTypeStr=Inherit: Same as input
  Kp6 : Gain  Gain=Kd  SampleTime=Ts  SaturateOnIntegerOverflow=on  OutDataTypeStr=Inherit: Same as input  ParamDataTypeStr=Inherit: Same as input
  Saturation2 : Saturate  UpperLimit=UpperLimit  LowerLimit=LowerLimit  SampleTime=Ts
  Sum6 : Sum  Inputs=+++  SampleTime=Ts  SaturateOnIntegerOverflow=on  InputSameDT=on  OutDataTypeStr=Inherit: Same as first input
  Zero-Order Hold : ZeroOrderHold  SampleTime=Ts
  Out : Outport  SampleTime=Ts  InitialOutput=0
  wires:
  Saturation2/1 -> Out/1
  Error/1 -> Kp4/1, Kp5/1, Kp6/1
  Sum6/1 -> Saturation2/1
  Kp5/1 -> Discrete-Time Integrator/1
  Kp6/1 -> "Derivative "/1
  Kp4/1 -> Zero-Order Hold/1
  Discrete-Time Integrator/1 -> Sum6/2
  "Derivative "/1 -> Sum6/3
  Zero-Order Hold/1 -> Sum6/1

== system off_grid_NPC/DC Regulator/Controller/DC Voltage Regulator/Discrete PI Controller ==
  note: Discrete PID Controller
  note: Pierre Giroux, Gilbert Sybille
      | Power System Simulation Laboratory
      | IREQ, Hydro-Quebc
  Error : Inport  SampleTime=Ts
  Discrete-Time Integrator : DiscreteIntegrator  InitialCondition=Init  SampleTime=Ts  LimitOutput=on  UpperSaturationLimit=UpperLimit  LowerSaturationLimit=LowerLimit  ICPrevOutput=DiscIntNeverNeededParam  ICPrevScaledInput=DiscIntNeverNeededParam
  Kp4 : Gain  Gain=Kp  SampleTime=Ts  SaturateOnIntegerOverflow=on  OutDataTypeStr=Inherit: Same as input  ParamDataTypeStr=Inherit: Same as input
  Kp5 : Gain  Gain=Ki  SampleTime=Ts  SaturateOnIntegerOverflow=on  OutDataTypeStr=Inherit: Same as input  ParamDataTypeStr=Inherit: Same as input
  Saturation2 : Saturate  UpperLimit=UpperLimit  LowerLimit=LowerLimit  SampleTime=Ts
  Sum6 : Sum  SampleTime=Ts  SaturateOnIntegerOverflow=on  InputSameDT=on  OutDataTypeStr=Inherit: Same as first input
  Zero-Order Hold : ZeroOrderHold  SampleTime=Ts
  Out : Outport  SampleTime=Ts  InitialOutput=0
  wires:
  Zero-Order Hold/1 -> Sum6/1
  Saturation2/1 -> Out/1
  Discrete-Time Integrator/1 -> Sum6/2
  Kp4/1 -> Zero-Order Hold/1
  Kp5/1 -> Discrete-Time Integrator/1
  Sum6/1 -> Saturation2/1
  Error/1 -> Kp5/1, Kp4/1
